simulink library "Aerodynamic"  (R2016a)
settings: Solver=ode45  StartTime=0.0  StopTime=10.0  RelTol=1e-3
values from neighbouring files (symbols this model uses):
  b = 21    [initACFT_high.m]
  c = 2.5    [initACFT_high.m]
  CD0 = 0.0281    [initACFT_high.m]
  CD_alpha = 0.5157    [initACFT_high.m]
  CD_elev = 0.0178    [initACFT_high.m]
  CL0 = 0.209    [initACFT_high.m]
  Cl_ail = -0.0453    [initACFT_high.m]
  CL_alpha = 8.7491    [initACFT_high.m]
  CL_AlphaDot = 1.27    [initACFT_high.m]
  Cl_beta = -0.1352    [initACFT_high.m]
  CL_elev = 0.5380    (= 0.538)    [initACFT_high.m]
  Cl_p = -0.45    [initACFT_high.m]
  CL_q = 4.14    [initACFT_high.m]
  Cl_r = 0.100    (= 0.1)    [initACFT_high.m]
  Cl_rud = 0.0333    [initACFT_high.m]
  Cm0 = 0.000    (= 0)    [initACFT_high.m]
  Cm_alpha = -2.4351    [initACFT_high.m]
  Cm_AlphaDot = -4.53    [initACFT_high.m]
  Cm_elev = -1.9079    [initACFT_high.m]
  Cm_q = -37.6    [initACFT_high.m]
  Cn_ail = -8.5944e-04    (= -0.00085944)    [initACFT_high.m]
  Cn_beta = 0.1478    [initACFT_high.m]
  Cn_p = -0.114    [initACFT_high.m]
  Cn_r = -0.15    [initACFT_high.m]
  Cn_rud = -0.1100    (= -0.11)    [initACFT_high.m]
  CY_ail = 0    [initACFT_high.m]
  CY_beta = -1.2777    [initACFT_high.m]
  CY_p = 0.300    (= 0.3)    [initACFT_high.m]
  CY_r = 0.910    (= 0.91)    [initACFT_high.m]
  CY_rud = 0.4343    [initACFT_high.m]
  S = 45    [initACFT_high.m]
  y_cg = 0    [initACFT_high.m]
  z_cg = -0.4    [initACFT_high.m]
settings Model: Creator=bruno  LastModifiedBy=bruno
settings DataIOCC: LimitDataPoints=on
settings DebuggingCC: AllowSymbolicDim=off

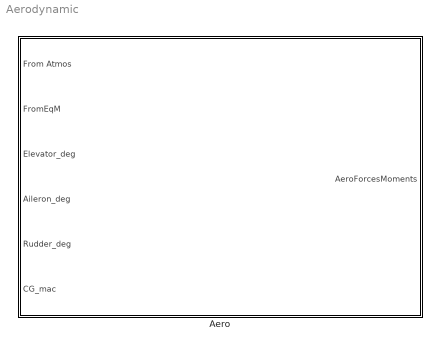
== system Aerodynamic ==
  Aero : Subsystem

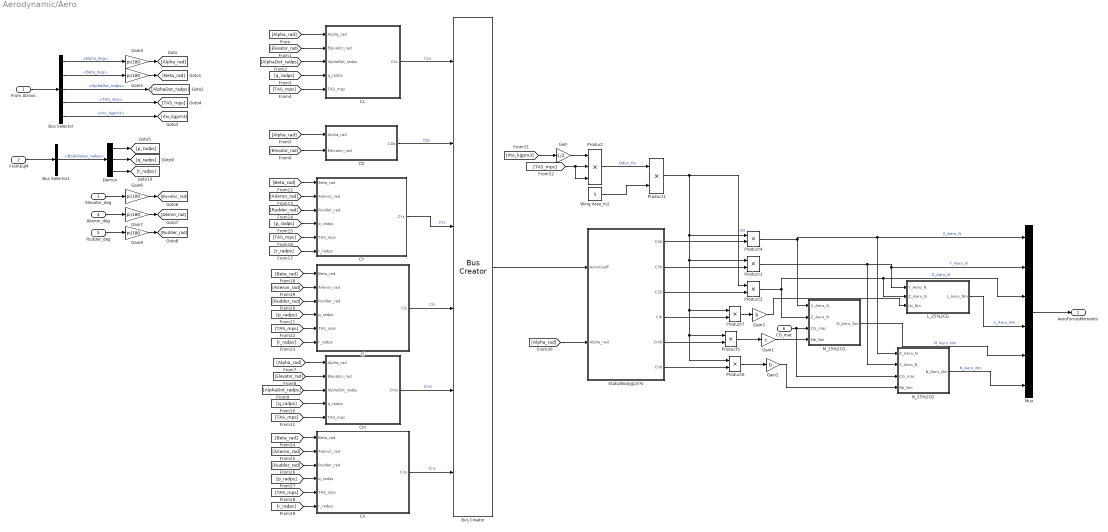
== system Aerodynamic/Aero ==
  From Atmos : Inport
  FromEqM : Inport  Port=2
  Elevator_deg : Inport  Port=3
  Aileron_deg : Inport  Port=4
  Rudder_deg : Inport  Port=5
  CG_mac : Inport  Port=6
  Bus Creator : BusCreator  Inputs=6
  Bus Selector : BusSelector  OutputSignals=Alpha_deg,Beta_deg,AlphaDot_radps,TAS_mps,rho_kgpm3
  Bus Selector1 : BusSelector  OutputSignals=BodyRates_radps
  CD : Subsystem
  CL : Subsystem
  CY : Subsystem
  Cl : Subsystem
  Cm : Subsystem
  Cn : Subsystem
  Demux : Demux  Outputs=3
  Gain : Gain  Gain=1/2
  Gain1 : Gain  Gain=c
  Gain2 : Gain  Gain=b
  Gain3 : Gain  Gain=b
  Gain{4..8} (5 alike) : Gain  Gain=pi/180
  L_25%2CG : Subsystem
  M_25%2CG : Subsystem
  Mux : Mux  Inputs=6
  N_25%2CG : Subsystem
  Product : Product  Inputs=3
  Product{1..7} (7 alike) : Product
  Stab2Body@25% : Subsystem
  Wing Area_m2 : Constant  Value=S
  AeroForcesMoments : Outport
  wires:
  Bus Selector1/1 -> Demux/1  "<BodyRates_radps>"
  FromEqM/1 -> Bus Selector1/1
  Bus Selector/1 -> Gain4/1  "<Alpha_deg>"
  From Atmos/1 -> Bus Selector/1
  [AlphaDot_radps] -> CL/3(AlphaDot_radps)
  [TAS_mps] -> CL/5(TAS_mps)
  Demux/3 -> [r_radps]
  Gain6/1 -> [Elevator_rad]
  Demux/1 -> [p_radps]
  Demux/2 -> [q_radps]
  Aileron_deg/1 -> Gain7/1
  Gain7/1 -> [Aileron_rad]
  Bus Selector/2 -> Gain5/1  "<Beta_deg>"
  [q_radps] -> CL/4(q_radps)
  [Alpha_rad] -> CD/1(Alpha_rad)
  Gain8/1 -> [Rudder_rad]
  [Elevator_rad] -> CD/2(Elevator_rad)
  [Alpha_rad] -> CL/1(Alpha_rad)
  Elevator_deg/1 -> Gain6/1
  [Elevator_rad] -> CL/2(Elevator_rad)
  [Alpha_rad] -> Cm/1(Alpha_rad)
  [Elevator_rad] -> Cm/2(Elevator_rad)
  Bus Selector/3 -> [AlphaDot_radps]  "<AlphaDot_radps>"
  Rudder_deg/1 -> Gain8/1
  Gain4/1 -> [Alpha_rad]
  Gain5/1 -> [Beta_rad]
  Mux/1 -> AeroForcesMoments/1
  [p_radps] -> CY/4(p_radps)
  Stab2Body@25%/2(CYb) -> Product3/2
  [p_radps] -> Cl/4(p_radps)
  Gain1/1 -> M_25%2CG/4(Mb_Nm)
  [Beta_rad] -> Cl/1(Beta_rad)
  [Beta_rad] -> Cn/1(Beta_rad)
  [Rudder_rad] -> CY/3(Rudder_rad)
  [Beta_rad] -> CY/1(Beta_rad)
  [r_radps] -> CY/6(r_radps)
  Wing Area_m2/1 -> Product1/2
  Cl/1(Cls) -> Bus Creator/4  "Cls"
  Stab2Body@25%/1(CXb) -> Product4/2
  Gain2/1 -> N_25%2CG/4(Nb_Nm)
  Product1/1 -> Product2/1, Product3/1, Product7/1, Product6/1, Product5/1, Product4/1  "QS"
  Stab2Body@25%/6(Cnb) -> Product6/2
  [TAS_mps] -> Cn/5(TAS_mps)
  CD/1(CDs) -> Bus Creator/2  "CDs"
  Product2/1 -> Mux/3, L_25%2CG/2(Z_Aero_N), M_25%2CG/2(Z_Aero_N)  "Z_Aero_N"
  [r_radps] -> Cn/6(r_radps)
  Bus Creator/1 -> Stab2Body@25%/1(AeroCoeff)
  [Rudder_rad] -> Cn/3(Rudder_rad)
  Stab2Body@25%/4(Clb) -> Product7/2
  Product7/1 -> Gain3/1
  [rho_kgpm3] -> Gain/1
  [Aileron_rad] -> Cl/2(Aileron_rad)
  Product3/1 -> Mux/2, L_25%2CG/1(Y_Aero_N), N_25%2CG/2(Y_Aero_N)  "Y_Aero_N"
  [TAS_mps] -> CY/5(TAS_mps)
  [TAS_mps] -> Product/3, Product/2
  Stab2Body@25%/3(CZb) -> Product2/2
  [TAS_mps] -> Cm/5(TAS_mps)
  Gain/1 -> Product/1
  Stab2Body@25%/5(Cmb) -> Product5/2
  [r_radps] -> Cl/6(r_radps)
  [Rudder_rad] -> Cl/3(Rudder_rad)
  CY/1(CYs) -> Bus Creator/3  "CYs"
  M_25%2CG/1(M_Aero_Nm) -> Mux/5  "M_Aero_Nm"
  Product6/1 -> Gain2/1
  Gain3/1 -> L_25%2CG/3(Lb_Nm)
  Cm/1(Cms) -> Bus Creator/5  "Cms"
  [Aileron_rad] -> CY/2(Aileron_rad)
  L_25%2CG/1(L_Aero_Nm) -> Mux/4  "L_Aero_Nm"
  CL/1(CLs) -> Bus Creator/1  "CLs"
  [TAS_mps] -> Cl/5(TAS_mps)
  Cn/1(Cns) -> Bus Creator/6  "Cns"
  [Alpha_rad] -> Stab2Body@25%/2(Alpha_rad)
  Product4/1 -> Mux/1, N_25%2CG/1(X_Aero_N), M_25%2CG/1(X_Aero_N)  "X_Aero_N"
  CG_mac/1 -> N_25%2CG/3(CG_mac), M_25%2CG/3(CG_mac)
  [AlphaDot_radps] -> Cm/3(AlphaDot_radps)
  [q_radps] -> Cm/4(q_radps)
  Product5/1 -> Gain1/1
  [p_radps] -> Cn/4(p_radps)
  [Aileron_rad] -> Cn/2(Aileron_rad)
  Product/1 -> Product1/1  "Qdyn_Pa"
  N_25%2CG/1(N_Aero_Nm) -> Mux/6  "N_Aero_Nm"
  Bus Selector/4 -> [TAS_mps]  "<TAS_mps>"
  Bus Selector/5 -> [rho_kgpm3]  "<rho_kgpm3>"

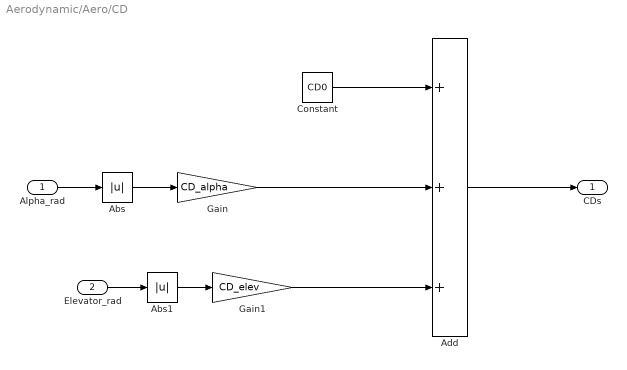
== system Aerodynamic/Aero/CD ==
  Alpha_rad : Inport
  Elevator_rad : Inport  Port=2
  Abs : Abs
  Abs1 : Abs
  Add : Sum  Inputs=+++
  Constant : Constant  Value=CD0
  Gain : Gain  Gain=CD_alpha
  Gain1 : Gain  Gain=CD_elev
  CDs : Outport
  wires:
  Abs1/1 -> Gain1/1
  Gain1/1 -> Add/3
  Abs/1 -> Gain/1
  Constant/1 -> Add/1
  Elevator_rad/1 -> Abs1/1
  Add/1 -> CDs/1
  Alpha_rad/1 -> Abs/1
  Gain/1 -> Add/2

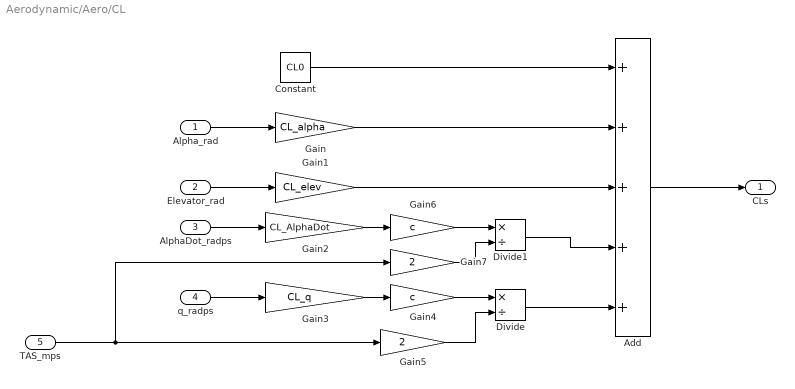
== system Aerodynamic/Aero/CL ==
  Alpha_rad : Inport
  Elevator_rad : Inport  Port=2
  AlphaDot_radps : Inport  Port=3
  q_radps : Inport  Port=4
  TAS_mps : Inport  Port=5
  Add : Sum  Inputs=+++++
  Constant : Constant  Value=CL0
  Divide : Product  Inputs=*/
  Divide1 : Product  Inputs=*/
  Gain : Gain  Gain=CL_alpha
  Gain1 : Gain  Gain=CL_elev
  Gain2 : Gain  Gain=CL_AlphaDot
  Gain3 : Gain  Gain=CL_q
  Gain4 : Gain  Gain=c
  Gain5 : Gain  Gain=2
  Gain6 : Gain  Gain=c
  Gain7 : Gain  Gain=2
  CLs : Outport
  wires:
  Divide1/1 -> Add/4
  Gain7/1 -> Divide1/2
  Gain6/1 -> Divide1/1
  Gain2/1 -> Gain6/1
  Divide/1 -> Add/5
  Gain5/1 -> Divide/2
  TAS_mps/1 -> Gain5/1, Gain7/1
  Gain4/1 -> Divide/1
  Gain3/1 -> Gain4/1
  Add/1 -> CLs/1
  Alpha_rad/1 -> Gain/1
  Gain1/1 -> Add/3
  Constant/1 -> Add/1
  Gain/1 -> Add/2
  q_radps/1 -> Gain3/1
  Elevator_rad/1 -> Gain1/1
  AlphaDot_radps/1 -> Gain2/1

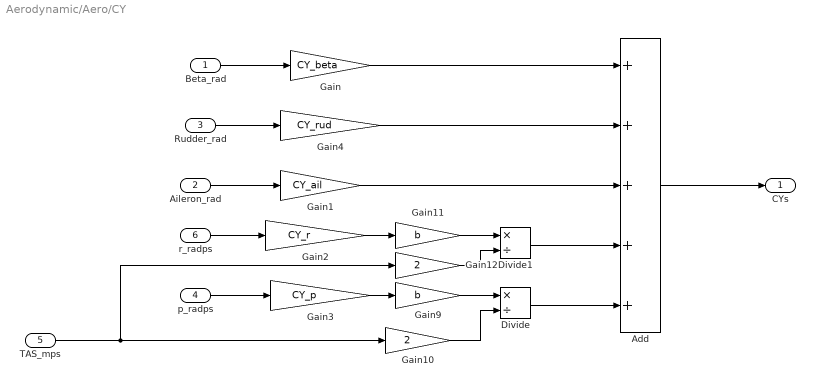
== system Aerodynamic/Aero/CY ==
  Beta_rad : Inport
  Aileron_rad : Inport  Port=2
  Rudder_rad : Inport  Port=3
  p_radps : Inport  Port=4
  TAS_mps : Inport  Port=5
  r_radps : Inport  Port=6
  Add : Sum  Inputs=+++++
  Divide : Product  Inputs=*/
  Divide1 : Product  Inputs=*/
  Gain : Gain  Gain=CY_beta
  Gain1 : Gain  Gain=CY_ail
  Gain10 : Gain  Gain=2
  Gain11 : Gain  Gain=b
  Gain12 : Gain  Gain=2
  Gain2 : Gain  Gain=CY_r
  Gain3 : Gain  Gain=CY_p
  Gain4 : Gain  Gain=CY_rud
  Gain9 : Gain  Gain=b
  CYs : Outport
  wires:
  r_radps/1 -> Gain2/1
  Gain4/1 -> Add/2
  Rudder_rad/1 -> Gain4/1
  Gain/1 -> Add/1
  Divide1/1 -> Add/4
  Gain2/1 -> Gain11/1
  Gain9/1 -> Divide/1
  Gain1/1 -> Add/3
  Gain10/1 -> Divide/2
  Gain12/1 -> Divide1/2
  Gain11/1 -> Divide1/1
  Add/1 -> CYs/1
  Divide/1 -> Add/5
  TAS_mps/1 -> Gain10/1, Gain12/1
  Beta_rad/1 -> Gain/1
  Gain3/1 -> Gain9/1
  p_radps/1 -> Gain3/1
  Aileron_rad/1 -> Gain1/1

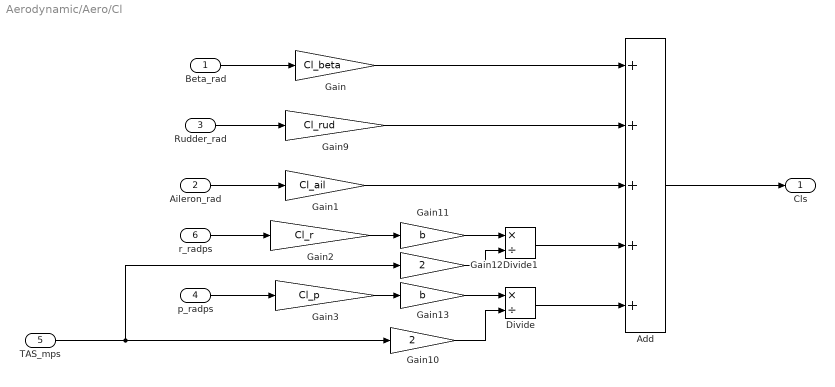
== system Aerodynamic/Aero/Cl ==
  Beta_rad : Inport
  Aileron_rad : Inport  Port=2
  Rudder_rad : Inport  Port=3
  p_radps : Inport  Port=4
  TAS_mps : Inport  Port=5
  r_radps : Inport  Port=6
  Add : Sum  Inputs=+++++
  Divide : Product  Inputs=*/
  Divide1 : Product  Inputs=*/
  Gain : Gain  Gain=Cl_beta
  Gain1 : Gain  Gain=Cl_ail
  Gain10 : Gain  Gain=2
  Gain11 : Gain  Gain=b
  Gain12 : Gain  Gain=2
  Gain13 : Gain  Gain=b
  Gain2 : Gain  Gain=Cl_r
  Gain3 : Gain  Gain=Cl_p
  Gain9 : Gain  Gain=Cl_rud
  Cls : Outport
  wires:
  Gain13/1 -> Divide/1
  Divide/1 -> Add/5
  Divide1/1 -> Add/4
  Gain2/1 -> Gain11/1
  Gain9/1 -> Add/2
  Gain12/1 -> Divide1/2
  Gain10/1 -> Divide/2
  Rudder_rad/1 -> Gain9/1
  Add/1 -> Cls/1
  Gain/1 -> Add/1
  Gain11/1 -> Divide1/1
  Gain1/1 -> Add/3
  r_radps/1 -> Gain2/1
  TAS_mps/1 -> Gain10/1, Gain12/1
  Beta_rad/1 -> Gain/1
  Gain3/1 -> Gain13/1
  p_radps/1 -> Gain3/1
  Aileron_rad/1 -> Gain1/1

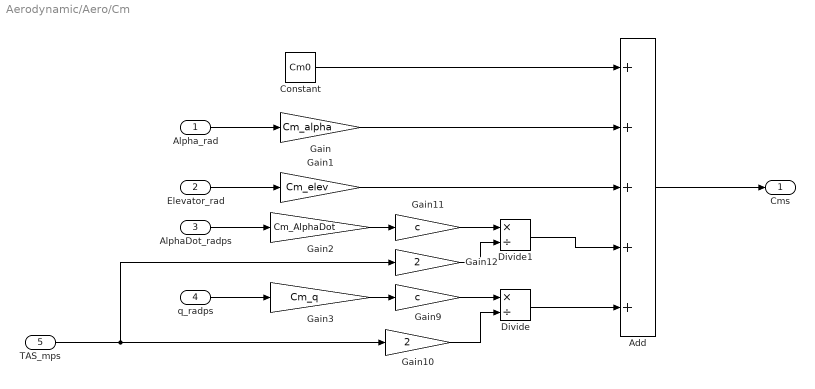
== system Aerodynamic/Aero/Cm ==
  Alpha_rad : Inport
  Elevator_rad : Inport  Port=2
  AlphaDot_radps : Inport  Port=3
  q_radps : Inport  Port=4
  TAS_mps : Inport  Port=5
  Add : Sum  Inputs=+++++
  Constant : Constant  Value=Cm0
  Divide : Product  Inputs=*/
  Divide1 : Product  Inputs=*/
  Gain : Gain  Gain=Cm_alpha
  Gain1 : Gain  Gain=Cm_elev
  Gain10 : Gain  Gain=2
  Gain11 : Gain  Gain=c
  Gain12 : Gain  Gain=2
  Gain2 : Gain  Gain=Cm_AlphaDot
  Gain3 : Gain  Gain=Cm_q
  Gain9 : Gain  Gain=c
  Cms : Outport
  wires:
  Gain10/1 -> Divide/2
  Divide1/1 -> Add/4
  Gain11/1 -> Divide1/1
  Gain12/1 -> Divide1/2
  Gain2/1 -> Gain11/1
  Divide/1 -> Add/5
  Gain1/1 -> Add/3
  Constant/1 -> Add/1
  q_radps/1 -> Gain3/1
  TAS_mps/1 -> Gain10/1, Gain12/1
  Gain9/1 -> Divide/1
  Gain3/1 -> Gain9/1
  Add/1 -> Cms/1
  Alpha_rad/1 -> Gain/1
  Gain/1 -> Add/2
  Elevator_rad/1 -> Gain1/1
  AlphaDot_radps/1 -> Gain2/1

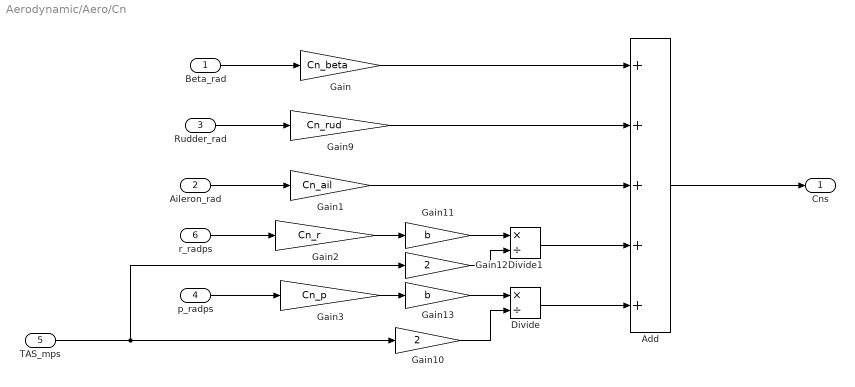
== system Aerodynamic/Aero/Cn ==
  Beta_rad : Inport
  Aileron_rad : Inport  Port=2
  Rudder_rad : Inport  Port=3
  p_radps : Inport  Port=4
  TAS_mps : Inport  Port=5
  r_radps : Inport  Port=6
  Add : Sum  Inputs=+++++
  Divide : Product  Inputs=*/
  Divide1 : Product  Inputs=*/
  Gain : Gain  Gain=Cn_beta
  Gain1 : Gain  Gain=Cn_ail
  Gain10 : Gain  Gain=2
  Gain11 : Gain  Gain=b
  Gain12 : Gain  Gain=2
  Gain13 : Gain  Gain=b
  Gain2 : Gain  Gain=Cn_r
  Gain3 : Gain  Gain=Cn_p
  Gain9 : Gain  Gain=Cn_rud
  Cns : Outport
  wires:
  Divide/1 -> Add/5
  Divide1/1 -> Add/4
  Gain9/1 -> Add/2
  Gain2/1 -> Gain11/1
  Gain13/1 -> Divide/1
  Gain10/1 -> Divide/2
  Rudder_rad/1 -> Gain9/1
  Gain12/1 -> Divide1/2
  Gain11/1 -> Divide1/1
  Gain1/1 -> Add/3
  r_radps/1 -> Gain2/1
  TAS_mps/1 -> Gain10/1, Gain12/1
  Aileron_rad/1 -> Gain1/1
  Beta_rad/1 -> Gain/1
  Gain3/1 -> Gain13/1
  Add/1 -> Cns/1
  p_radps/1 -> Gain3/1
  Gain/1 -> Add/1

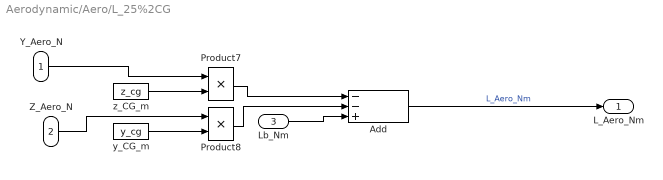
== system Aerodynamic/Aero/L_25%2CG ==
  Y_Aero_N : Inport
  Z_Aero_N : Inport  Port=2
  Lb_Nm : Inport  Port=3
  Add : Sum  Inputs=--+
  Product7 : Product
  Product8 : Product
  y_CG_m : Constant  Value=y_cg
  z_CG_m : Constant  Value=z_cg
  L_Aero_Nm : Outport
  wires:
  z_CG_m/1 -> Product7/2
  Product8/1 -> Add/2
  Product7/1 -> Add/1
  Lb_Nm/1 -> Add/3
  Add/1 -> L_Aero_Nm/1  "L_Aero_Nm"
  y_CG_m/1 -> Product8/2
  Y_Aero_N/1 -> Product7/1
  Z_Aero_N/1 -> Product8/1

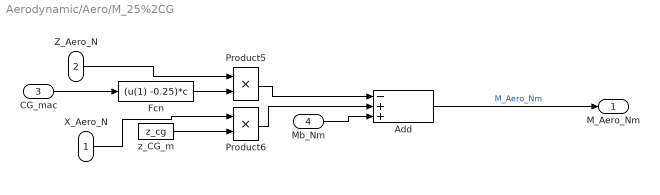
== system Aerodynamic/Aero/M_25%2CG ==
  X_Aero_N : Inport
  Z_Aero_N : Inport  Port=2
  CG_mac : Inport  Port=3
  Mb_Nm : Inport  Port=4
  Add : Sum  Inputs=-++
  Fcn : Fcn  Expr=(u(1) -0.25)*c
  Product5 : Product
  Product6 : Product
  z_CG_m : Constant  Value=z_cg
  M_Aero_Nm : Outport
  wires:
  Mb_Nm/1 -> Add/3
  CG_mac/1 -> Fcn/1
  Fcn/1 -> Product5/2
  Product5/1 -> Add/1
  Z_Aero_N/1 -> Product5/1
  X_Aero_N/1 -> Product6/1
  Add/1 -> M_Aero_Nm/1  "M_Aero_Nm"
  Product6/1 -> Add/2
  z_CG_m/1 -> Product6/2

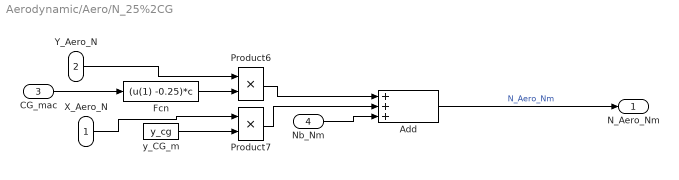
== system Aerodynamic/Aero/N_25%2CG ==
  X_Aero_N : Inport
  Y_Aero_N : Inport  Port=2
  CG_mac : Inport  Port=3
  Nb_Nm : Inport  Port=4
  Add : Sum  Inputs=+++
  Fcn : Fcn  Expr=(u(1) -0.25)*c
  Product6 : Product
  Product7 : Product
  y_CG_m : Constant  Value=y_cg
  N_Aero_Nm : Outport
  wires:
  Y_Aero_N/1 -> Product6/1
  CG_mac/1 -> Fcn/1
  X_Aero_N/1 -> Product7/1
  Product6/1 -> Add/1
  Fcn/1 -> Product6/2
  Nb_Nm/1 -> Add/3
  Add/1 -> N_Aero_Nm/1  "N_Aero_Nm"
  y_CG_m/1 -> Product7/2
  Product7/1 -> Add/2

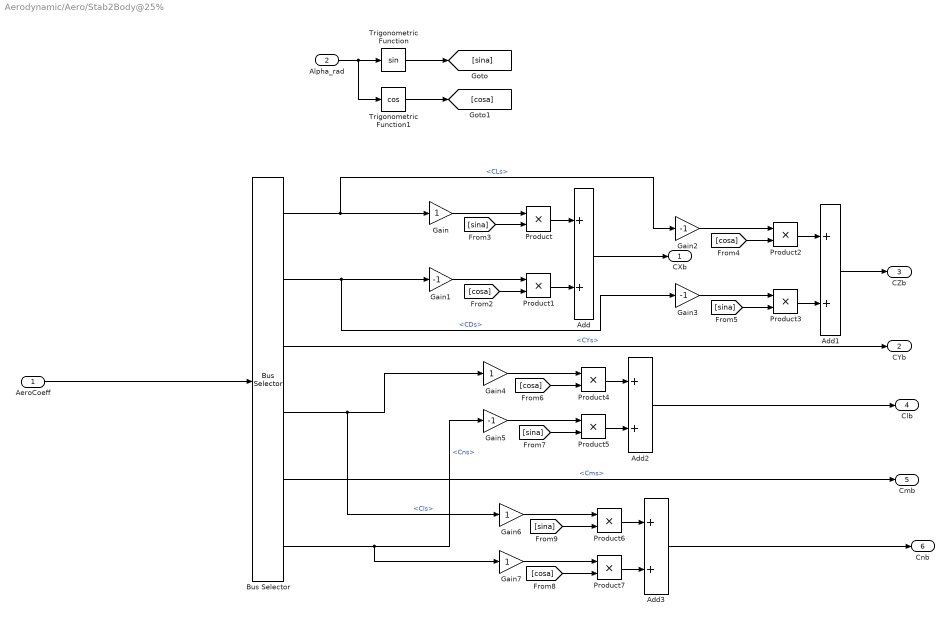
== system Aerodynamic/Aero/Stab2Body@25% ==
  AeroCoeff : Inport
  Alpha_rad : Inport  Port=2
  Add{,1..3} (4 alike) : Sum
  Bus Selector : BusSelector  OutputSignals=CLs,CDs,CYs,Cls,Cms,Cns
  Gain{,4,6..7} (4 alike) : Gain
  Gain{1..3,5} (4 alike) : Gain  Gain=-1
  Product{,1..7} (8 alike) : Product
  Trigonometric Function : Trigonometry
  Trigonometric Function1 : Trigonometry  Operator=cos
  CXb : Outport
  CYb : Outport  Port=2
  CZb : Outport  Port=3
  Clb : Outport  Port=4
  Cmb : Outport  Port=5
  Cnb : Outport  Port=6
  wires:
  [cosa] -> Product7/2
  Product7/1 -> Add3/2
  Add3/1 -> Cnb/1
  Product6/1 -> Add3/1
  Gain7/1 -> Product7/1
  Gain6/1 -> Product6/1
  [sina] -> Product6/2
  [sina] -> Product5/2
  Bus Selector/6 -> Gain5/1, Gain7/1  "<Cns>"
  Bus Selector/4 -> Gain4/1, Gain6/1  "<Cls>"
  Product5/1 -> Add2/2
  Add2/1 -> Clb/1
  Product4/1 -> Add2/1
  Gain5/1 -> Product5/1
  Gain4/1 -> Product4/1
  [cosa] -> Product4/2
  Bus Selector/5 -> Cmb/1  "<Cms>"
  Bus Selector/3 -> CYb/1  "<CYs>"
  [cosa] -> Product2/2
  [sina] -> Product3/2
  Add1/1 -> CZb/1
  Product2/1 -> Add1/1
  Product3/1 -> Add1/2
  Gain3/1 -> Product3/1
  Gain2/1 -> Product2/1
  Add/1 -> CXb/1
  Product/1 -> Add/1
  Product1/1 -> Add/2
  Gain1/1 -> Product1/1
  Bus Selector/2 -> Gain1/1, Gain3/1  "<CDs>"
  [cosa] -> Product1/2
  Gain/1 -> Product/1
  Bus Selector/1 -> Gain/1, Gain2/1  "<CLs>"
  [sina] -> Product/2
  Trigonometric Function1/1 -> [cosa]
  Trigonometric Function/1 -> [sina]
  Alpha_rad/1 -> Trigonometric Function/1, Trigonometric Function1/1
  AeroCoeff/1 -> Bus Selector/1
